simulink model "simulation_commande_sliding_mode_2"  (R2020a)
settings: Solver=VariableStepAuto  StartTime=0.0  StopTime=10.0  RelTol=1e-3
values from neighbouring files (symbols this model uses):
  a = 1    [Adap.m]    (also in Adaptive_control_Non_linear.m = 2; HOSM.m; projet_AAV.m; sys.m)
  b = 2    [Adaptive_Control_Linear.m]    (also in Adaptive_control_Non_linear.m; HOSM.m = 1; feedback-integrator.m = 3; mini_projet.m = 3)
settings Model: Creator=lenovo  LastModifiedBy=lenovo
settings SolverCC: ZeroCrossAlgorithm=Adaptive
settings DebuggingCC: IgnoredZcDiagnostic=none

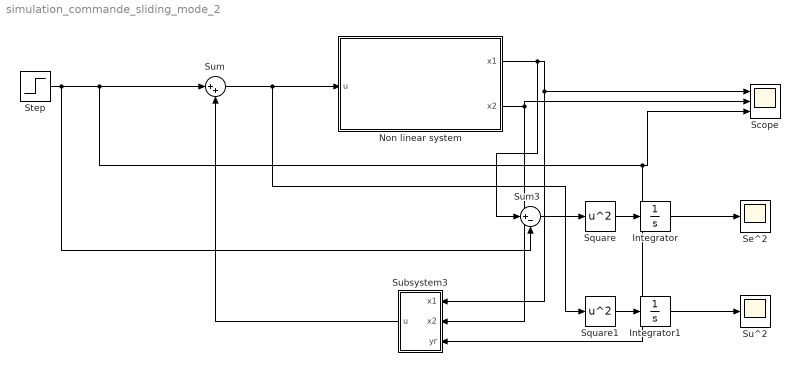
== system simulation_commande_sliding_mode_2 ==
  Integrator : Integrator
  Integrator1 : Integrator
  Non linear system : Subsystem
  Scope : Scope  NumInputPorts=3
  Se^2 : Scope
  Square : Math  Operator=square  SaturateOnIntegerOverflow=on
  Square1 : Math  Operator=square  SaturateOnIntegerOverflow=on
  Step : Step  Time=0  SampleTime=0
  Su^2 : Scope
  Subsystem3 : Subsystem
  Sum : Sum  Inputs=|++
  Sum3 : Sum  Inputs=|+-
  wires:
  Non linear system/2(x2) -> Subsystem3/2(x2), Scope/2
  Step/1 -> Sum3/2, Subsystem3/3(yr), Scope/3, Sum/1
  Subsystem3/1(u) -> Sum/2
  Sum3/1 -> Square/1
  Square/1 -> Integrator/1
  Integrator/1 -> Se^2/1
  Sum/1 -> Square1/1, Non linear system/1(u)
  Integrator1/1 -> Su^2/1
  Square1/1 -> Integrator1/1
  Non linear system/1(x1) -> Sum3/1, Scope/1, Subsystem3/1(x1)

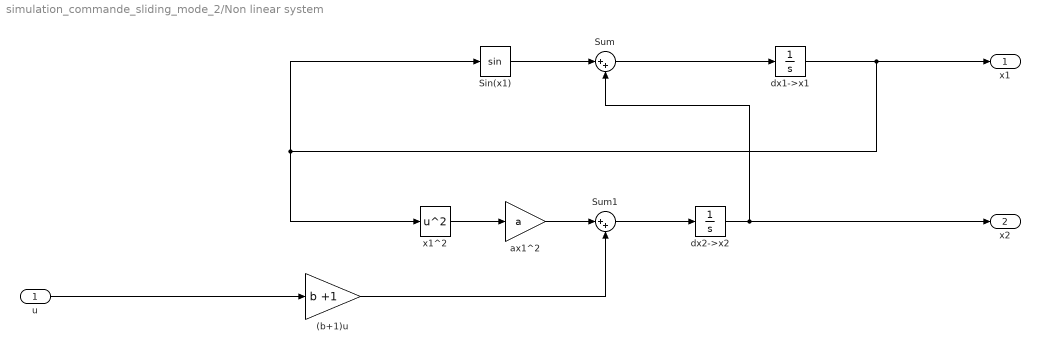
== system simulation_commande_sliding_mode_2/Non linear system ==
  u : Inport
  (b+1)u : Gain  Gain=b +1
  Sin(x1) : Trigonometry
  Sum : Sum  Inputs=|++
  Sum1 : Sum  Inputs=|++
  ax1^2 : Gain  Gain=a
  dx1->x1 : Integrator
  dx2->x2 : Integrator
  x1^2 : Math  Operator=square  SaturateOnIntegerOverflow=on
  x1 : Outport
  x2 : Outport  Port=2
  wires:
  (b+1)u/1 -> Sum1/2
  dx2->x2/1 -> x2/1, Sum/2
  u/1 -> (b+1)u/1
  ax1^2/1 -> Sum1/1
  dx1->x1/1 -> Sin(x1)/1, x1^2/1, x1/1
  Sin(x1)/1 -> Sum/1
  x1^2/1 -> ax1^2/1
  Sum1/1 -> dx2->x2/1
  Sum/1 -> dx1->x1/1

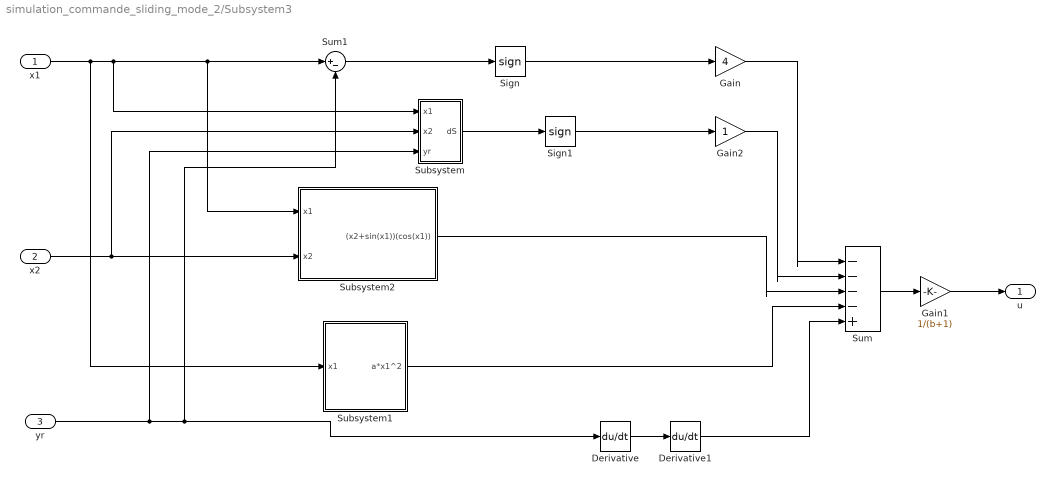
== system simulation_commande_sliding_mode_2/Subsystem3 ==
  x1 : Inport
  x2 : Inport  Port=2
  yr : Inport  Port=3
  Derivative : Derivative
  Derivative1 : Derivative
  Gain : Gain  Gain=4
  Gain1 : Gain  Gain=1/(b+1)
  Gain2 : Gain
  Sign : Signum
  Sign1 : Signum
  Subsystem : Subsystem
  Subsystem1 : Subsystem
  Subsystem2 : Subsystem
  Sum : Sum  Inputs=|----+
  Sum1 : Sum  Inputs=|+-
  u : Outport
  wires:
  yr/1 -> Subsystem/3(yr), Derivative/1, Sum1/2
  x1/1 -> Subsystem1/1("x1 "), Subsystem/1(x1), Sum1/1, Subsystem2/1("x1 ")
  Gain/1 -> Sum/1
  Subsystem/1(dS) -> Sign1/1
  Sign1/1 -> Gain2/1
  x2/1 -> Subsystem/2(x2), Subsystem2/2(x2)
  Sum/1 -> Gain1/1
  Sign/1 -> Gain/1
  Derivative1/1 -> Sum/5
  Gain1/1 -> u/1
  Derivative/1 -> Derivative1/1
  Gain2/1 -> Sum/2
  Subsystem1/1(a*x1^2) -> Sum/4
  Sum1/1 -> Sign/1
  Subsystem2/1((x2+sin(x1))(cos(x1))) -> Sum/3

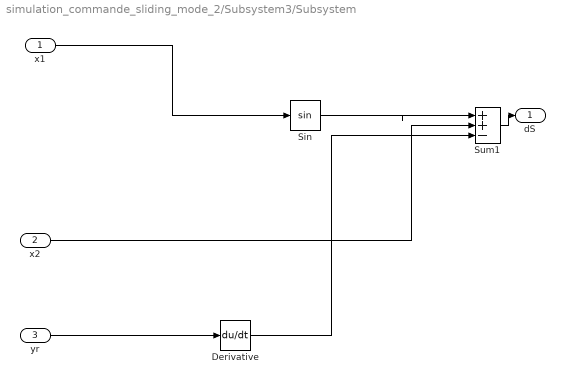
== system simulation_commande_sliding_mode_2/Subsystem3/Subsystem ==
  x1 : Inport
  x2 : Inport  Port=2
  yr : Inport  Port=3
  Derivative : Derivative
  Sin : Trigonometry
  Sum1 : Sum  Inputs=|++-
  dS : Outport
  wires:
  Sin/1 -> Sum1/1
  x1/1 -> Sin/1
  Sum1/1 -> dS/1
  x2/1 -> Sum1/2
  yr/1 -> Derivative/1
  Derivative/1 -> Sum1/3

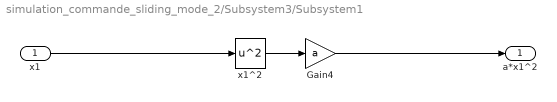
== system simulation_commande_sliding_mode_2/Subsystem3/Subsystem1 ==
  "x1 " : Inport
  Gain4 : Gain  Gain=a
  x1^2 : Math  Operator=square  SaturateOnIntegerOverflow=on
  a*x1^2 : Outport
  wires:
  x1^2/1 -> Gain4/1
  Gain4/1 -> a*x1^2/1
  "x1 "/1 -> x1^2/1

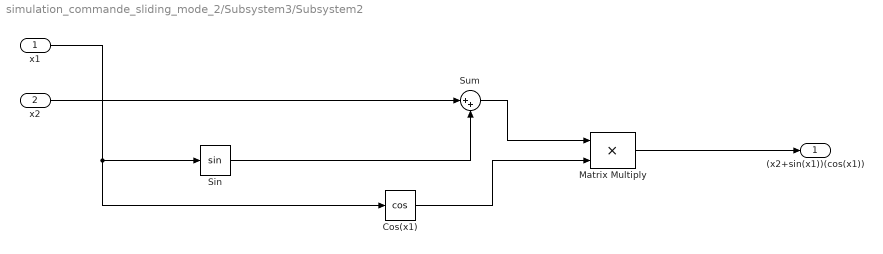
== system simulation_commande_sliding_mode_2/Subsystem3/Subsystem2 ==
  "x1 " : Inport
  x2 : Inport  Port=2
  Cos(x1) : Trigonometry  Operator=cos
  Matrix Multiply : Product
  Sin : Trigonometry
  Sum : Sum  Inputs=|++
  (x2+sin(x1))(cos(x1)) : Outport
  wires:
  x2/1 -> Sum/1
  Matrix Multiply/1 -> (x2+sin(x1))(cos(x1))/1
  Sum/1 -> Matrix Multiply/1
  Cos(x1)/1 -> Matrix Multiply/2
  "x1 "/1 -> Cos(x1)/1, Sin/1
  Sin/1 -> Sum/2
